simulink model "ModeloFuncion1"  (R2021a)
settings: Solver=VariableStepAuto  StartTime=0.0  StopTime=10.0  RelTol=1e-3
settings Model: Creator=Estudiante  LastModifiedBy=Estudiante

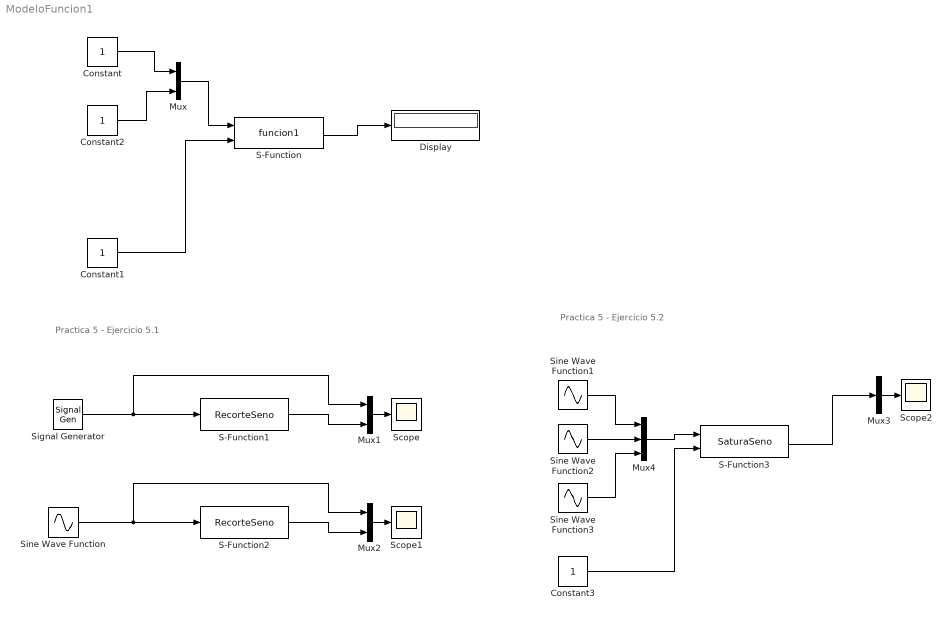
== system ModeloFuncion1 ==
  note: Practica 5 - Ejercicio 5.1
  note: Practica 5 - Ejercicio 5.2
  Constant{,1..3} (4 alike) : Constant
  Display : Display
  Mux : Mux  Inputs=2
  Mux1 : Mux  Inputs=2
  Mux2 : Mux  Inputs=2
  Mux3 : Mux  Inputs=1
  Mux4 : Mux  Inputs=3
  S-Function : S-Function  InitFcn=mex funcion1.c  FunctionName=funcion1  Parameters=10 10  SFunctionDeploymentMode=off  EnableBusSupport=off
  S-Function1 : S-Function  InitFcn=mex RecorteSeno.c  FunctionName=RecorteSeno  Parameters=3 -3  SFunctionDeploymentMode=off  EnableBusSupport=off
  S-Function2 : S-Function  InitFcn=mex RecorteSeno.c  FunctionName=RecorteSeno  Parameters=3 -3  SFunctionDeploymentMode=off  EnableBusSupport=off
  S-Function3 : S-Function  InitFcn=mex SaturaSeno.c  FunctionName=SaturaSeno  Parameters=0 0  SFunctionDeploymentMode=off  EnableBusSupport=off
  Scope : Scope
  Scope1 : Scope
  Scope2 : Scope
  Signal Generator : SignalGenerator  Amplitude=5  Units=rad/sec
  Sine Wave Function : Sin  Amplitude=4  SampleTime=0
  Sine Wave Function1 : Sin  Amplitude=4  SampleTime=0
  Sine Wave Function2 : Sin  Amplitude=4  Phase=pi/3  SampleTime=0
  Sine Wave Function3 : Sin  Amplitude=4  Phase=2*pi/3  SampleTime=0
  wires:
  S-Function/1 -> Display/1
  Constant1/1 -> S-Function/2
  Constant/1 -> Mux/1
  Mux/1 -> S-Function/1
  Constant2/1 -> Mux/2
  Signal Generator/1 -> Mux1/1, S-Function1/1
  Mux1/1 -> Scope/1
  S-Function1/1 -> Mux1/2
  S-Function2/1 -> Mux2/2
  Mux2/1 -> Scope1/1
  Sine Wave Function/1 -> S-Function2/1, Mux2/1
  Mux3/1 -> Scope2/1
  Sine Wave Function1/1 -> Mux4/1
  Sine Wave Function2/1 -> Mux4/2
  Sine Wave Function3/1 -> Mux4/3
  Mux4/1 -> S-Function3/1
  Constant3/1 -> S-Function3/2
  S-Function3/1 -> Mux3/1
